simulink model "PVAndBatteryIntegratedPlantForBlackStart_SPS"  (R2024b)
settings: Solver=FixedStepAuto  StartTime=0.0  StopTime=tsim  FixedStep=Ts  RelTol=1e-9  AbsTol=1e-7
InitFcn:
  | %% Black Start Sequence
  | t0 = 0; % Battery IBR initial time
  | t1 = 0.5; % PV IBR initial time
  | t2 = 0.8; % Two IBR sync time
  | t3 = 1.2; % Additional motor load connect
  | t4 = 1.5; % Grid reconnection
  | tsim = 3.0; % Total simulation time
  | 
  | %% System Parameters
  | Vdc = 400;
  | Vnom = 100;
  | Prated = 10000;
  | Qrated = 0;
  | Srated = sqrt(Prated^2+Qrated^2);
  | wnom = 2*pi*60;
  | fnom = 60;
  | 
  | %% VOC Parameters
  | kv = Vnom;
  | ki = 3*Vnom/Srated;
  | Vminpu = 0.95;
  | dwmax = 0.5*2*pi;
  | trisemax = 0.1;
  | 
  | C = 1/sqrt(2)/Vminpu^2/dwmax;
  | L = 1/C/wnom^2;
  | tau = C/kv/ki;
  | epsilon = sqrt(L/C);
  | ksy = 3/2/trisemax;
  | 
  | V_voc_1 = 0;
  | V_voc_2 = 0;
  | 
  | %% Filter Parameters
  | Rf = 0.05;
  | Lf = 500e-6;
  | fsw = 10e3;
  | Ts = 1e-6;
  | 
  | %% Load Parameters
  | Rl = 3*Vnom^2/Prated;
  | Rl1 = Rl;
  | Rl2 = 2*Rl;
  | Rl3 = 20*Rl;
  | 
  | %% DCDC Converter Parameters
  | Kp_V = 1;
  | Ki_V = 10;
  | Imax = 110;
  | Kp_I = 0.0001;
  | Ki_I = 1;
  | Vcmax = 1;
undefined symbols (not defined in the file): C_voc, L_voc, Ll, R_voc
libraries: spsThreePhaseVIMeasurementLib x8, eeTransforms x7, spsHalfBridgeConverterLib x6, spsThreePhaseBreakerLib x6, spsThreePhaseSeriesRLCBranchLib x5, spsControlledCurrentSourceLib x4, spsControlledVoltageSourceLib x4, spsParallelRLCBranchLib x4, spsCurrentMeasurementLib x3, spsVoltageMeasurementLib x3, spsGroundLib x3, spsPower3phInstantaneousLib x3
(part 2 of 2)

== system PVAndBatteryIntegratedPlantForBlackStart_SPS/PV Inverter /Inverter Control/VOC Control/Subsystem/rotate ==
  deltai : Inport
  Demux : Demux  Outputs=2
  Gain : Gain  Gain=-1
  Mux : Mux  Inputs=2
  u : Outport
  wires:
  Demux/1 -> Mux/2
  Gain/1 -> Mux/1
  Demux/2 -> Gain/1
  Mux/1 -> u/1
  deltai/1 -> Demux/1
